simulink model "ControlPI_AntiWindUp"  (R2020a)
settings: Solver=VariableStepAuto  StartTime=0.0  StopTime=2000  RelTol=1e-3
settings Model: Creator=RogerCondori  LastModifiedBy=RogerCondori

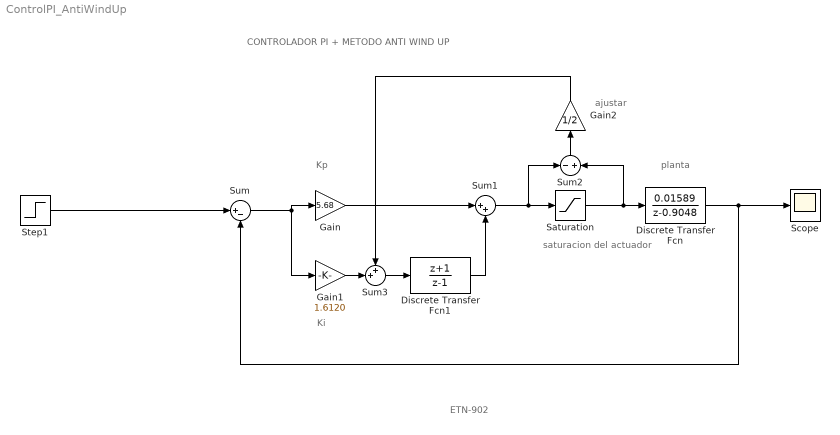
== system ControlPI_AntiWindUp ==
  note: ajustar
  note: Kp
  note: Ki
  note: saturacion
      | del actuador
  note: planta
  note: CONTROLADOR PI + METODO ANTI WIND UP
  note: ETN-902
  Discrete Transfer Fcn : DiscreteTransferFcn  Numerator=[0.01589]  Denominator=[1 -0.9048]
  Discrete Transfer Fcn1 : DiscreteTransferFcn  Numerator=[1 1]  Denominator=[1 -1]  InitialStates=1
  Gain : Gain  Gain=5.68
  Gain1 : Gain  Gain=1.6120
  Gain2 : Gain  Gain=1/2
  Saturation : Saturate  UpperLimit=40  LowerLimit=0
  Scope : Scope
  Step1 : Step  Time=0  SampleTime=0
  Sum : Sum  Inputs=|+-
  Sum1 : Sum  Inputs=|++
  Sum2 : Sum  Inputs=-|+
  Sum3 : Sum  Inputs=++|
  wires:
  Sum/1 -> Gain1/1, Gain/1
  Discrete Transfer Fcn/1 -> Scope/1, Sum/2
  Step1/1 -> Sum/1
  Gain/1 -> Sum1/1
  Discrete Transfer Fcn1/1 -> Sum1/2
  Sum1/1 -> Sum2/1, Saturation/1
  Saturation/1 -> Sum2/2, Discrete Transfer Fcn/1
  Sum3/1 -> Discrete Transfer Fcn1/1
  Gain1/1 -> Sum3/2
  Gain2/1 -> Sum3/1
  Sum2/1 -> Gain2/1
